simulink model "B4_subsystem"  (R2018b)
settings: Solver=ode45  StartTime=0.0  StopTime=10.0  MaxStep=0.01  RelTol=1e-3  EnableMultiTasking=on
values from neighbouring files (symbols this model uses):
  c = 3    [B2_create_variables.m]    (also in B2_create_variablesA.m = 2)
  k = 0.2    [B2_create_variables.m]    (also in B2_create_variablesA.m = 0.5)
  m = 1    [B2_create_variables.m]    (also in B2_create_variablesA.m)
  v0 = 0    [B2_create_variables.m]    (also in B2_create_variablesA.m)
  y0 = 3.0    (= 3)    [B2_create_variables.m]    (also in B2_create_variablesA.m)
settings Model: Creator=Reichl  LastModifiedBy=Reichl
settings DataIOCC: LimitDataPoints=on  SaveFormat=Array  SignalLoggingSaveFormat=ModelDataLogs
settings OptimizationCC: ExpressionDepthLimit=2147483647  LifeSpan=inf
settings DebuggingCC: UnderspecifiedInitializationDetection=Classic  MergeDetectMultiDrivingBlocksExec=none  SolverPrmCheckMsg=warning  FcnCallInpInsideContextMsg=warning  StateNameClashWarn=warning  SFUnexpectedBacktrackingDiag=warning  SFNoUnconditionalDefaultTransitionDiag=warning  SFExecutionAtInitializationDiag=none
settings HardwareCC: ProdBitPerPointer=32  ProdBitPerSizeT=32  ProdBitPerPtrDiffT=32  ProdLargestAtomicFloat=None  ProdIntDivRoundTo=Undefined  ProdEndianess=Unspecified  ProdWordSize=32  ProdHWDeviceType=32-bit Generic
settings ModelReferenceCC: PropagateSignalLabelsOutOfModel=off
settings SFSimCC: SimUseLocalCustomCode=off
settings RTWCC: RTWUseLocalCustomCode=off
settings CodeAppCC: StateflowObjectComments=on
settings GRTTargetCC: TargetLangStandard=C89/C90 (ANSI)  GeneratePreprocessorConditionals=Disable all  CombineOutputUpdateFcns=off  GRTInterface=on
settings ConfigComp: CovMetricSettings=dw  CovHtmlReporting=on  CovSaveCumulativeToWorkspaceVar=on  CovSaveSingleToWorkspaceVar=on  CovExternalEMLEnable=off

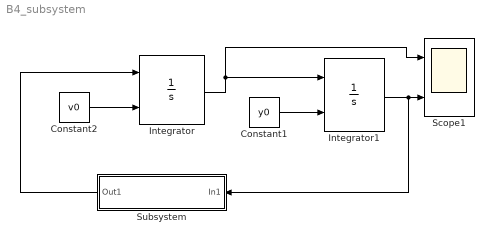
== system B4_subsystem ==
  Constant1 : Constant  Value=y0
  Constant2 : Constant  Value=v0
  Integrator : Integrator  InitialConditionSource=external
  Integrator1 : Integrator  InitialConditionSource=external  InitialCondition=3
  Scope1 : Scope  NumInputPorts=2
  Subsystem : Subsystem
  wires:
  Integrator/1 -> Integrator1/1, Scope1/1
  Constant2/1 -> Integrator/2
  Constant1/1 -> Integrator1/2
  Integrator1/1 -> Scope1/2, Subsystem/1(In1)
  Subsystem/1(Out1) -> Integrator/1

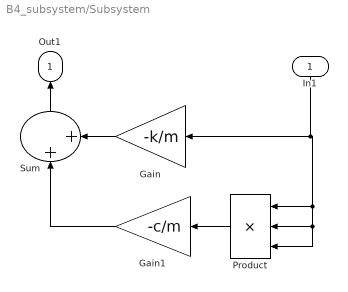
== system B4_subsystem/Subsystem ==
  In1 : Inport
  Gain : Gain  Gain=-k/m
  Gain1 : Gain  Gain=-c/m
  Product : Product  Inputs=***  RndMeth=Zero
  Sum : Sum  Inputs=|++
  Out1 : Outport
  wires:
  Gain/1 -> Sum/2
  Product/1 -> Gain1/1
  Sum/1 -> Out1/1
  Gain1/1 -> Sum/1
  In1/1 -> Gain/1, Product/3, Product/2, Product/1
